simulink model "suspension_estimator_OL_CL"  (R2021b)
settings: Solver=VariableStepAuto  StartTime=0.0  StopTime=80  RelTol=1e-6  EnableMultiTasking=on
values from neighbouring files (symbols this model uses):
  A = [0   1 ... (first row only)    [DC_motor_example_LQR_v2.m]    (also in First_example_LQR.m = 1; IP.m = [0     0     1      0; ip_example.m = [ 0          0        1         0; suspension_estimator.m = [      0            1           0           0)
  B = [0 ... (first row only)    [DC_motor_example_LQR_v2.m]    (also in First_example_LQR.m = 1; IP.m = [0; 0; 3.7778; -12.3862]; ip_example.m = [ 0; suspension_estimator.m = [ 0)
  B1 = [0 ... (first row only)    [suspension_estimator.m]
  C = [1 0]    [DC_motor_example_LQR_v2.m]    (also in First_example_LQR.m = 1; ip_example.m = [1  0  0  0; suspension_estimator.m = [0  0  1  0]; transmission_zeros_example1.m = [1 0 1 0)
  K = lqr(A,B,Q,R)    [DC_motor_example_LQR_v2.m]    (also in First_example_LQR.m = K_vector(j); ip_example.m = acker(A,B,cl_poles); suspension_estimator.m = acker(A,B,cl_poles); two_tanks_tracking_controller.m = place(A,B,cl_poles))
  L = acker(A',C',poles_estimator)'    [suspension_estimator.m]
  x0 = 10    [First_example_LQR.m]    (also in ex1.m = z(1:length(A)); ip_example.m = [0  15*pi/180 0 0 ]; suspension_estimator.m = [0.2 0 0.1 0]'; transmission_zeros_example1.m = V(1:4,3))
settings Model: Creator=magudelo  LastModifiedBy=yz
settings SolverCC: AlgebraicLoopSolver=TrustRegion
settings DataIOCC: LimitDataPoints=on  ReturnWorkspaceOutputs=off
settings OptimizationCC: LifeSpan=inf
settings DebuggingCC: AllowSymbolicDim=off  SFUnexpectedBacktrackingDiag=warning  SFNoUnconditionalDefaultTransitionDiag=warning  SFExecutionAtInitializationDiag=none  SFMachineParentedDataDiag=warning  ArithmeticOperatorsInVariantConditions=warning
settings ModelReferenceCC: PropagateSignalLabelsOutOfModel=off
settings SFSimCC: SimUseLocalCustomCode=off  CustomCodeUndefinedFunction=UseInterfaceOnly
settings RTWCC: RTWUseLocalCustomCode=off
settings CodeAppCC: StateflowObjectComments=on
settings GRTTargetCC: TargetLangStandard=C89/C90 (ANSI)
settings ConfigComp: CovMetricSettings=dw  CovSaveCumulativeToWorkspaceVar=on  CovSaveSingleToWorkspaceVar=on  CovExternalEMLEnable=off

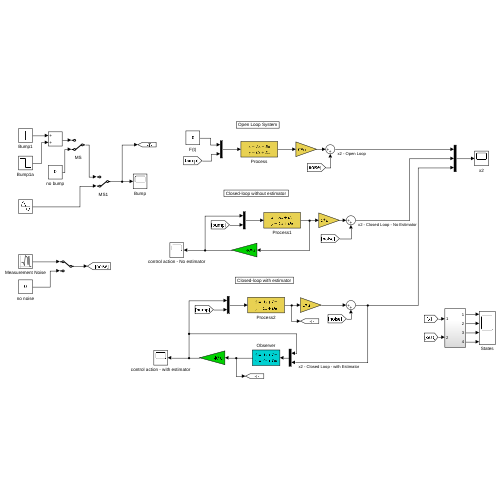
[thumbnail: Simulink's stored preview of the top-level diagram]
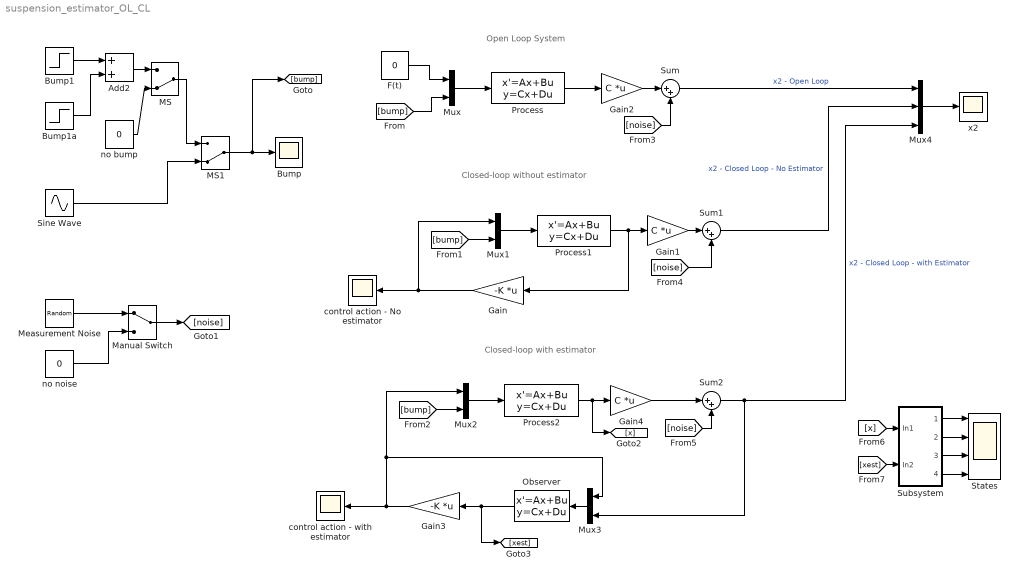
== system suspension_estimator_OL_CL ==
  note: Closed-loop without estimator
  note: Open Loop System
  note: Closed-loop with estimator
  Add2 : Sum
  Bump : Scope
  Bump1 : Step  Time=25  After=0.2  SampleTime=0
  Bump1a : Step  Time=25.5  After=-0.2  SampleTime=0
  F(t) : Constant  Value=0
  Gain : Gain  Gain=-K  Multiplication=Matrix(K*u)
  Gain1 : Gain  Gain=C  Multiplication=Matrix(K*u)
  Gain2 : Gain  Gain=C  Multiplication=Matrix(K*u)
  Gain3 : Gain  Gain=-K  Multiplication=Matrix(K*u)
  Gain4 : Gain  Gain=C  Multiplication=Matrix(K*u)
  MS : ManualSwitch  CurrentSetting=0
  MS1 : ManualSwitch  CurrentSetting=0
  Manual Switch : ManualSwitch
  Measurement Noise : RandomNumber  Variance=1e-6  SampleTime=0.001
  Mux{,1..3} (4 alike) : Mux  Inputs=2
  Mux4 : Mux  Inputs=3
  Observer : StateSpace  A=A-L*C  B=[B L]  C=eye(4,4)  D=zeros(4,2)  InitialCondition=[0 0 0 0]
  Process : StateSpace  A=A  B=[B B1]  C=eye(4)  D=zeros(4,2)  InitialCondition=x0
  Process1 : StateSpace  A=A  B=[B B1]  C=eye(4)  D=zeros(4,2)  InitialCondition=x0
  Process2 : StateSpace  A=A  B=[B B1]  C=eye(4)  D=zeros(4,2)  InitialCondition=x0
  Sine Wave : Sin  SampleTime=0
  States : Scope  NumInputPorts=4
  Subsystem : Subsystem
  Sum : Sum  Inputs=|++
  Sum1 : Sum  Inputs=|++
  Sum2 : Sum  Inputs=|++
  control action - No estimator : Scope
  control action - with estimator : Scope
  no bump : Constant  Value=0
  no noise : Constant  Value=0
  x2 : Scope
  wires:
  Process/1 -> Gain2/1
  Bump1/1 -> Add2/1
  Bump1a/1 -> Add2/2
  Mux/1 -> Process/1
  F(t)/1 -> Mux/1
  Process1/1 -> Gain/1, Gain1/1
  Mux1/1 -> Process1/1
  [bump] -> Mux/2
  [bump] -> Mux1/2
  Gain/1 -> control action - No estimator/1, Mux1/1
  Process2/1 -> [x], Gain4/1
  Mux2/1 -> Process2/1
  [bump] -> Mux2/2
  Gain3/1 -> Mux2/1, Mux3/1, control action - with estimator/1
  Observer/1 -> [xest], Gain3/1
  Mux3/1 -> Observer/1
  Manual Switch/1 -> [noise]
  Measurement Noise/1 -> Manual Switch/1
  no noise/1 -> Manual Switch/2
  Gain2/1 -> Sum/1
  Sum/1 -> Mux4/1  "x2 - Open Loop"
  [noise] -> Sum/2
  Gain1/1 -> Sum1/1
  Sum1/1 -> Mux4/2  "x2 - Closed Loop - No Estimator"
  [noise] -> Sum1/2
  Gain4/1 -> Sum2/1
  [noise] -> Sum2/2
  Sum2/1 -> Mux4/3, Mux3/2  "x2 - Closed Loop - with Estimator"
  Mux4/1 -> x2/1
  [x] -> Subsystem/1(In1)
  [xest] -> Subsystem/2(In2)
  Subsystem/1(Out1) -> States/1
  Subsystem/2(Out2) -> States/2
  Subsystem/3(Out3) -> States/3
  Subsystem/4(Out4) -> States/4
  Add2/1 -> MS/1
  no bump/1 -> MS/2
  MS/1 -> MS1/1
  MS1/1 -> [bump], Bump/1
  Sine Wave/1 -> MS1/2

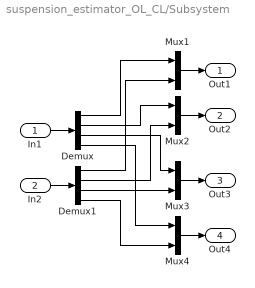
== system suspension_estimator_OL_CL/Subsystem ==
  In1 : Inport
  In2 : Inport  Port=2
  Demux : Demux
  Demux1 : Demux
  Mux{1..4} (4 alike) : Mux  Inputs=2
  Out1 : Outport
  Out2 : Outport  Port=2
  Out3 : Outport  Port=3
  Out4 : Outport  Port=4
  wires:
  Demux/1 -> Mux1/1
  Demux1/1 -> Mux1/2
  Demux/2 -> Mux2/1
  Demux1/2 -> Mux2/2
  Demux/3 -> Mux3/1
  Demux1/3 -> Mux3/2
  Demux/4 -> Mux4/1
  Demux1/4 -> Mux4/2
  Mux1/1 -> Out1/1
  Mux2/1 -> Out2/1
  In1/1 -> Demux/1
  Mux3/1 -> Out3/1
  In2/1 -> Demux1/1
  Mux4/1 -> Out4/1
